simulink model "clv3d"  (Simulink 3.00)
settings: Solver=ode45  SolverMode=SingleTasking  StartTime=0.0  StopTime=40  RelTol=1e-3  AbsTol=1e-6
undefined symbols (not defined in the file or in its folder): sfunxyz
settings Model: ExternalInput=[]  SaveTime=off  SaveOutput=off  InitialState=[]  IntegerOverflowMsg=none  RTWOptions="-aEnforceIntegerDowncast=1 -aFoldNonRolledExpr=1 -aInlineInvariantSignals=1 -aInlineParameters=0 -aLocalBlockOutputs=1 -aRollThreshold=5 -aZeroInternalMemoryAtStartup=1 -aZeroExternalMemoryAtStartup=1 -aInitFltsAndDblsToZero=1 -aGenerateReport=0 -aGenCodeOnly=0 -aRTWVerbose=1 -aIncludeHyperlinkInReport=0 -aLaunchReport=0 -aForceParamTrailComments=0 -aGenerateComments=1 -aIgnoreCustomStorageClasses=1 -aIncHierarchyInIds=0 -aMaxRTWIdLen=31 -aShowEliminatedStatements=0 -aPrefixModelToSubsysFcnNames=1 -aIncDataTypeInIds=0 -aInsertBlockDesc=0 -aSimulinkBlockComments=1 -aInlinedPrmAccess=\"Literals\"  -aSuppressErrorStatus=0 -aModelReferenceCompliant=1 -aSupportNonInlinedSFcns=1 -aSupportContinuousTime=1 -aSupportComplex=1 -aSupportNonFinite=1 -aSupportAbsoluteTime=1 -aTargetFcnLib=\"ansi_tfl_tmw.mat\" -aMultiInstanceERTCode=0 -aLogVarNameModifier=\"rt_\" -aIsPILTarget=0 -aCombineOutputUpdateFcns=0 -aGenerateASAP2=0 -aGenerateSampleERTMain=0 -aGenerateFullHeader=1 -aUtilityFuncGeneration=\"Auto\" -aIncludeFileDelimiter=\"Auto\" -aIncludeMdlTerminateFcn=1 -aPurelyIntegerCode=0 -aERTCustomFileBanners=0 -aRTWCAPIStates=0 -aRTWCAPIParams=0 -aRTWCAPISignals=0 -aMatFileLogging=1 -aGenFloatMathFcnCalls=\"ANSI_C\" -aExtModeMexFile=\"ext_comm\" -aExtModeTransport=0 -aExtModeStaticAllocSize=1000000 -aExtModeTesting=0 -aExtModeStaticAlloc=0 -aExtMode=0  -aInitFltsAndDblsToZero=1 -aInitFltsAndDblsToZero=1 -aInitFltsAndDblsToZero=1"  Creator=The MathWorks Inc.  LastModifiedBy=campa

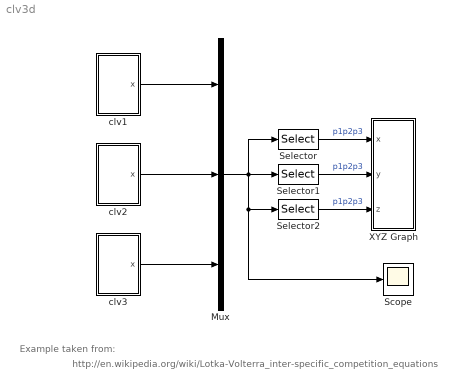
== system clv3d ==
  note: Example taken from:
  note: http://en.wikipedia.org/wiki/Lotka-Volterra_inter-specific_competition_equations
  Mux : Mux  Inputs=[4 4 4]
  Scope : Scope
      settings: TimeRange=40  YMin=0  YMax=0.8  SaveToWorkspace=off  SaveName=ScopeData
  Selector : Selector  Elements=[1 5 9]  InputPortWidth=12
  Selector1 : Selector  Elements=[2 6 10]  InputPortWidth=12
  Selector2 : Selector  Elements=[3 7 11]  InputPortWidth=12
  XYZ Graph : Subsystem  LoadFcn=sfunxyz([],[],[],'LoadBlock')  StartFcn=sfunxyz([],[],[],'Start')  StopFcn=sfunxyz([],[],[],'Stop')  mask(XYZ multiscope){np=3, xlim=[-1 1], ylim=[-1 1], zlim=[0 1], cp=[1 2 3], gd=on, st=0.01}
      mask prompts: np "Number of lines"; xlim "[xmin xmax]"; ylim "[ymin ymax]"; zlim "[zmin zmax]"; cp "Camera position (use [0 0 1] for 2D XY view)"; gd "Grid"; st "Sample time:"
      mask help:
      | Multidimensional XYZ scope using MATLAB graph window.
      |    X,Y,Z coordinates are respectively the first,second, and third input.
      |    Enter the number of lines, the XYZ ranges, the camera position,
      |    and the sampling time, as mask parameters.
      settings: CopyFcn=sfunxyz([],[],[],'CopyBlock')  DeleteFcn=sfunxyz([],[],[],'DeleteBlock')  NameChangeFcn=sfunxyz([],[],[],'NameChange')
      mask Help:
      | This block can be used to explore limit cycles.
      |    Look at the m-file sfunxyz.m to see how it works.
      mask Display: plot([.05 .95 .95 .05 .05],[.45 .45 .95 .95 .45], 0.5+cos(0:0.1:2*pi)*0.3,0.7+sin(0:0.1:2*pi)*0.2)
  clv1 : Subsystem  mask(Competitive Lotka Volterra System){A=[1 1.09 1.52 0; 0 1 0.44 1.36; 2.33 0 1 1.47; 1.21 0.51 0.35 1], R=diag([1 0.72 1.53 1.27]), x0=[0.2 0.2 0.2 0.1]}
      mask prompts: x0 "Initial Condition"
      mask help:
      | This autonomous system represents the competitive lotka volterra system
      |  xdot =  Rx .* ( 1 - Ax)
      |  where each component of x represents a population,
      |  A is an interaction matrix, and R is a diagonal "growth rate" matrix.
      |  Parameters and initial state can be selected from the mask.
      mask Help:
      | This autonomous system represents the competitive lotka volterra system
      |  <p>
      |  The system equations are:
      |  xdot =  Rx .* ( 1 - Ax)
      |  where each component of x represents a population,
      |  A is an interaction matrix, and R is a diagonal "growth rate" matrix.
      |  Parameters and initial state can be selected from the mask.
  clv2 : Subsystem  mask(Competitive Lotka Volterra System){A=[1 1.09 1.52 0; 0 1 0.44 1.36; 2.33 0 1 1.47; 1.21 0.51 0.35 1], R=diag([1 0.72 1.53 1.27]), x0=[0.2 0.2 0.2 0.2]}
      mask prompts: x0 "Initial Condition"
      mask help:
      | This autonomous system represents the competitive lotka volterra system
      |  xdot =  Rx .* ( 1 - Ax)
      |  where each component of x represents a population,
      |  A is an interaction matrix, and R is a diagonal "growth rate" matrix.
      |  Parameters and initial state can be selected from the mask.
      mask Help:
      | This autonomous system represents the competitive lotka volterra system
      |  <p>
      |  The system equations are:
      |  xdot =  Rx .* ( 1 - Ax)
      |  where each component of x represents a population,
      |  A is an interaction matrix, and R is a diagonal "growth rate" matrix.
      |  Parameters and initial state can be selected from the mask.
  clv3 : Subsystem  mask(Competitive Lotka Volterra System){A=[1 1.09 1.52 0; 0 1 0.44 1.36; 2.33 0 1 1.47; 1.21 0.51 0.35 1], R=diag([1 0.72 1.53 1.27]), x0=[0.2 0.2 0.2 0.3]}
      mask prompts: x0 "Initial Condition"
      mask help:
      | This autonomous system represents the competitive lotka volterra system
      |  xdot =  Rx .* ( 1 - Ax)
      |  where each component of x represents a population,
      |  A is an interaction matrix, and R is a diagonal "growth rate" matrix.
      |  Parameters and initial state can be selected from the mask.
      mask Help:
      | This autonomous system represents the competitive lotka volterra system
      |  <p>
      |  The system equations are:
      |  xdot =  Rx .* ( 1 - Ax)
      |  where each component of x represents a population,
      |  A is an interaction matrix, and R is a diagonal "growth rate" matrix.
      |  Parameters and initial state can be selected from the mask.
  wires:
  Mux/1 -> Selector1/1, Selector/1, Scope/1, Selector2/1
  Selector/1 -> XYZ Graph/1(x)  "p1p2p3"
  Selector1/1 -> XYZ Graph/2(y)  "p1p2p3"
  clv1/1(x) -> Mux/1
  clv2/1(x) -> Mux/2
  clv3/1(x) -> Mux/3
  Selector2/1 -> XYZ Graph/3(z)  "p1p2p3"

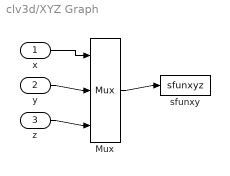
== system clv3d/XYZ Graph ==
  x : Inport  Port=1  PortWidth=-1  SampleTime=-1  DataType=auto
      settings: SignalType=auto
  y : Inport  Port=2  PortWidth=-1  SampleTime=-1  DataType=auto
      settings: SignalType=auto
  z : Inport  Port=3  PortWidth=-1  SampleTime=-1  DataType=auto
      settings: SignalType=auto
  Mux : Mux  Inputs=[np np np]
      settings: DisplayOption=none
  sfunxy : S-Function  FunctionName=sfunxyz  Parameters=[xlim ylim zlim],st,np,cp,gd  PortCounts=[]  SFunctionModules=''
  wires:
  z/1 -> Mux/3
  y/1 -> Mux/2
  x/1 -> Mux/1
  Mux/1 -> sfunxy/1

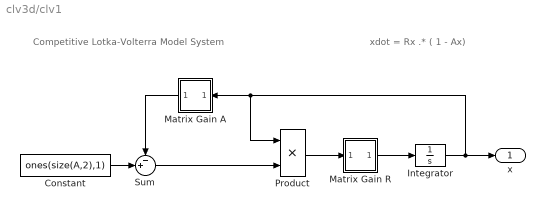
== system clv3d/clv1 ==
  note: Competitive Lotka-Volterra Model System
  note: xdot = Rx .* ( 1 - Ax)
  Constant : Constant  Value=ones(size(A,2),1)
  Integrator : Integrator  ExternalReset=none  InitialConditionSource=internal  InitialCondition=x0  LimitOutput=off  UpperSaturationLimit=inf  LowerSaturationLimit=-inf  ShowSaturationPort=off  ShowStatePort=off  AbsoluteTolerance=auto
  Matrix Gain A : Subsystem  Orientation=left  mask(Matrix Gain){K=A}
      mask prompts: K "Gain matrix:"
      mask help: Matrix Gain.
      mask Help: Multiplies input vector by entered matrix to produce output vector (y=Au).
      mask Display: disp('A')
  Matrix Gain R : Subsystem  mask(Matrix Gain){K=R}
      mask prompts: K "Gain matrix:"
      mask help: Matrix Gain.
      mask Help: Multiplies input vector by entered matrix to produce output vector (y=Au).
      mask Display: disp('R')
  Product : Product  Inputs=2  SaturateOnIntegerOverflow=on
  Sum : Sum  Inputs=-+|  SaturateOnIntegerOverflow=off
  x : Outport  Port=1
  wires:
  Constant/1 -> Sum/2
  Matrix Gain A/1(Out1) -> Sum/1
  Sum/1 -> Product/2
  Integrator/1 -> x/1, Product/1, Matrix Gain A/1(In1)
  Product/1 -> Matrix Gain R/1(In1)
  Matrix Gain R/1(Out1) -> Integrator/1

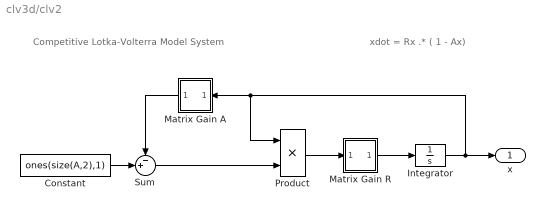
== system clv3d/clv2 ==
  note: xdot = Rx .* ( 1 - Ax)
  note: Competitive Lotka-Volterra Model System
  Constant : Constant  Value=ones(size(A,2),1)
  Integrator : Integrator  ExternalReset=none  InitialConditionSource=internal  InitialCondition=x0  LimitOutput=off  UpperSaturationLimit=inf  LowerSaturationLimit=-inf  ShowSaturationPort=off  ShowStatePort=off  AbsoluteTolerance=auto
  Matrix Gain A : Subsystem  Orientation=left  mask(Matrix Gain){K=A}
      mask prompts: K "Gain matrix:"
      mask help: Matrix Gain.
      mask Help: Multiplies input vector by entered matrix to produce output vector (y=Au).
      mask Display: disp('A')
  Matrix Gain R : Subsystem  mask(Matrix Gain){K=R}
      mask prompts: K "Gain matrix:"
      mask help: Matrix Gain.
      mask Help: Multiplies input vector by entered matrix to produce output vector (y=Au).
      mask Display: disp('R')
  Product : Product  Inputs=2  SaturateOnIntegerOverflow=on
  Sum : Sum  Inputs=-+|  SaturateOnIntegerOverflow=off
  x : Outport  Port=1
  wires:
  Matrix Gain R/1(Out1) -> Integrator/1
  Product/1 -> Matrix Gain R/1(In1)
  Integrator/1 -> Matrix Gain A/1(In1), Product/1, x/1
  Sum/1 -> Product/2
  Matrix Gain A/1(Out1) -> Sum/1
  Constant/1 -> Sum/2

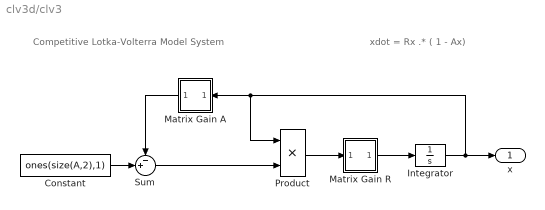
== system clv3d/clv3 ==
  note: Competitive Lotka-Volterra Model System
  note: xdot = Rx .* ( 1 - Ax)
  Constant : Constant  Value=ones(size(A,2),1)
  Integrator : Integrator  ExternalReset=none  InitialConditionSource=internal  InitialCondition=x0  LimitOutput=off  UpperSaturationLimit=inf  LowerSaturationLimit=-inf  ShowSaturationPort=off  ShowStatePort=off  AbsoluteTolerance=auto
  Matrix Gain A : Subsystem  Orientation=left  mask(Matrix Gain){K=A}
      mask prompts: K "Gain matrix:"
      mask help: Matrix Gain.
      mask Help: Multiplies input vector by entered matrix to produce output vector (y=Au).
      mask Display: disp('A')
  Matrix Gain R : Subsystem  mask(Matrix Gain){K=R}
      mask prompts: K "Gain matrix:"
      mask help: Matrix Gain.
      mask Help: Multiplies input vector by entered matrix to produce output vector (y=Au).
      mask Display: disp('R')
  Product : Product  Inputs=2  SaturateOnIntegerOverflow=on
  Sum : Sum  Inputs=-+|  SaturateOnIntegerOverflow=off
  x : Outport  Port=1
  wires:
  Constant/1 -> Sum/2
  Matrix Gain A/1(Out1) -> Sum/1
  Sum/1 -> Product/2
  Integrator/1 -> x/1, Product/1, Matrix Gain A/1(In1)
  Product/1 -> Matrix Gain R/1(In1)
  Matrix Gain R/1(Out1) -> Integrator/1

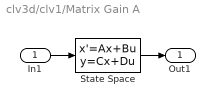
== system clv3d/clv1/Matrix Gain A ==
  In1 : Inport  Port=1  PortWidth=-1  SampleTime=-1  DataType=auto
      settings: SignalType=auto
  State Space : StateSpace  A=[]  B=[]  C=[]  D=K  X0=0
  Out1 : Outport  Port=1
  wires:
  In1/1 -> State Space/1
  State Space/1 -> Out1/1

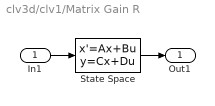
== system clv3d/clv1/Matrix Gain R ==
  In1 : Inport  Port=1  PortWidth=-1  SampleTime=-1  DataType=auto
      settings: SignalType=auto
  State Space : StateSpace  A=[]  B=[]  C=[]  D=K  X0=0
  Out1 : Outport  Port=1
  wires:
  State Space/1 -> Out1/1
  In1/1 -> State Space/1

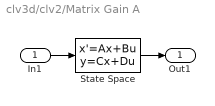
== system clv3d/clv2/Matrix Gain A ==
  In1 : Inport  Port=1  PortWidth=-1  SampleTime=-1  DataType=auto
      settings: SignalType=auto
  State Space : StateSpace  A=[]  B=[]  C=[]  D=K  X0=0
  Out1 : Outport  Port=1
  wires:
  State Space/1 -> Out1/1
  In1/1 -> State Space/1

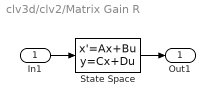
== system clv3d/clv2/Matrix Gain R ==
  In1 : Inport  Port=1  PortWidth=-1  SampleTime=-1  DataType=auto
      settings: SignalType=auto
  State Space : StateSpace  A=[]  B=[]  C=[]  D=K  X0=0
  Out1 : Outport  Port=1
  wires:
  In1/1 -> State Space/1
  State Space/1 -> Out1/1

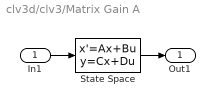
== system clv3d/clv3/Matrix Gain A ==
  In1 : Inport  Port=1  PortWidth=-1  SampleTime=-1  DataType=auto
      settings: SignalType=auto
  State Space : StateSpace  A=[]  B=[]  C=[]  D=K  X0=0
  Out1 : Outport  Port=1
  wires:
  In1/1 -> State Space/1
  State Space/1 -> Out1/1

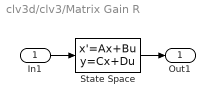
== system clv3d/clv3/Matrix Gain R ==
  In1 : Inport  Port=1  PortWidth=-1  SampleTime=-1  DataType=auto
      settings: SignalType=auto
  State Space : StateSpace  A=[]  B=[]  C=[]  D=K  X0=0
  Out1 : Outport  Port=1
  wires:
  State Space/1 -> Out1/1
  In1/1 -> State Space/1
